simulink model "ControladorContinuo"  (Simulink 7.9)
settings: Solver=ode5  StartTime=0.0  StopTime=inf  RelTol=1e-3
values from neighbouring files (symbols this model uses):
  a = [0  1  0; 0  0  1; -792900  -79150  -14.01]    [workspace.mat]
  b = [7.711 -167.9 63100]    [workspace.mat]
  c = [1 0 0]    [workspace.mat]
  h = [15.99 -79074.0199 -949681.481201]    [workspace.mat]
  ki = -23.6307990829    [workspace.mat]
  kp = [2.35890748821 0.000417540035136 2.98030004827e-05]    [workspace.mat]
  tm = 0.01    [workspace.mat]
undefined symbols (not defined in the file or in its folder): National_Instruments, PCI
libraries: rtwinlib x2, simulink x1
settings Model: Creator=oscar_mau.fernandez  LastModifiedBy=automatica  SimulationMode=external
settings HardwareCC: ProdIntDivRoundTo=Zero  ProdEndianess=LittleEndian  ProdHWDeviceType=Generic->32-bit x86 compatible
settings RTWCC: SystemTargetFile=rtwin.tlc  TemplateMakefile=rtwin.tmf  Description=Real-Time Windows Target  RetainRTWFile=on  ProcessScript=rtwin_make_rtw_hook  RTWCompilerOptimization=On
settings CodeAppCC: MaxIdLength=95
settings RTWinTargetCC: TargetLibSuffix=_rtwin.lib  TargetPreCompLibLocation=C:\Archivos de programa\MATLAB\R2012a\toolbox\rtw\targets\rtwin\lib\win32  CodeReplacementLibrary=ANSI_C  CodeExecutionProfiling=off  PortableWordSizes=off  RTWinDir=C:/ARCHIV~1/MATLAB/R2012a/toolbox/rtw/targets/rtwin  TargetArch=win32  RebuildAll=on

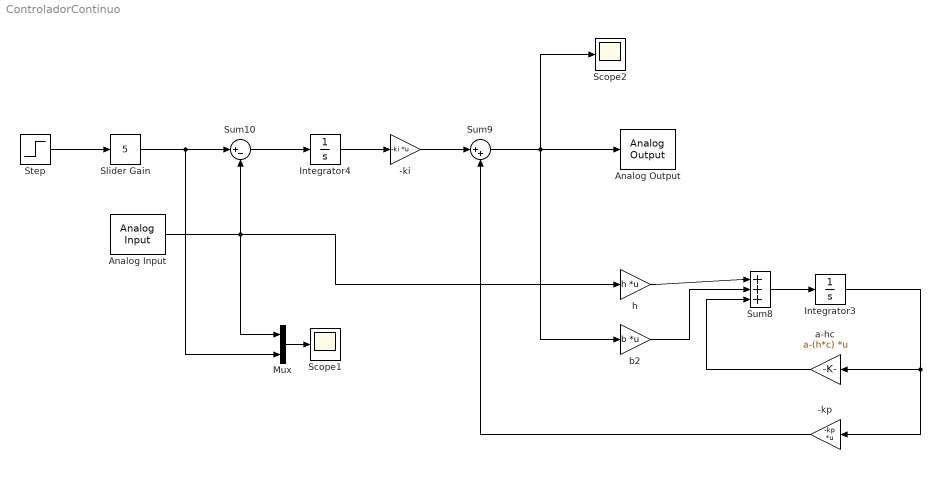
== system ControladorContinuo ==
  -ki : Gain  Gain=-ki  Multiplication=Matrix(K*u) (u vector)
  -kp : Gain  Gain=-kp  Multiplication=Matrix(K*u) (u vector)
  Analog Input : rtwinlib/Analog Input  SampleTime=tm  MaxMissedTicks=10  ShowMissedTicks=off  YieldWhenWaiting=off  DrvName=National_Instruments/PCI-6221  DrvAddress=4294967295  DrvOptions=[1 0 0 0 0]  Channels=1  RangeMode=1  VoltRange=2  DataType=1
      settings: AttributesFormatString=National Instruments\nPCI-6221 [auto]
  Analog Output : rtwinlib/Analog Output  SampleTime=tm  MaxMissedTicks=10  ShowMissedTicks=off  YieldWhenWaiting=off  DrvName=National_Instruments/PCI-6221  DrvAddress=4294967295  DrvOptions=[1 0 0 0 0]  Channels=1  RangeMode=1  VoltRange=1  InitialValue=0  FinalValue=5
      settings: AttributesFormatString=National Instruments\nPCI-6221 [auto]
  Integrator3 : Integrator
  Integrator4 : Integrator
  Mux : Mux  Inputs=2
  Scope1 : Scope
      settings: TimeRange=100  YMin=4.85  YMax=5.02
  Scope2 : Scope
      settings: TimeRange=100  YMin=5.85  YMax=6.8
  Slider Gain : simulink/Math Operations/Slider Gain  low=0  gain=5  high=5
  Step : Step  Time=0
  Sum10 : Sum  Inputs=|+-
  Sum8 : Sum  Inputs=|+++
  Sum9 : Sum  Inputs=|++
  a-hc : Gain  Gain=a-(h*c)  Multiplication=Matrix(K*u) (u vector)
  b2 : Gain  Gain=b  Multiplication=Matrix(K*u) (u vector)
  h : Gain  Gain=h  Multiplication=Matrix(K*u) (u vector)
  wires:
  h/1 -> Sum8/1
  b2/1 -> Sum8/2
  Sum8/1 -> Integrator3/1
  Integrator3/1 -> a-hc/1, -kp/1
  Sum9/1 -> Analog Output/1, b2/1, Scope2/1
  -ki/1 -> Sum9/1
  Integrator4/1 -> -ki/1
  Sum10/1 -> Integrator4/1
  -kp/1 -> Sum9/2
  Analog Input/1 -> Sum10/2, Mux/1, h/1
  Step/1 -> Slider Gain/1
  Mux/1 -> Scope1/1
  Slider Gain/1 -> Sum10/1, Mux/2
  a-hc/1 -> Sum8/3
